simulink model "BugE_v0_40_MAS_loads_reg"  (R2015b)
settings: Solver=FixedStepDiscrete  StartTime=0.0  StopTime=1370  FixedStep=sample_time  RelTol=1e-3
values from neighbouring files (symbols this model uses):
  AB_diode_dV = 0.9    [main_sync.m]
  air_density = 1.225    [main_sync.m]
  bus_ac_Pmax_abs = 240    [main_sync.m]
  bus_charger_Pmax = 1000    [main_sync.m]
  bus_load_Pmax_abs = 260    [main_sync.m]
  capInitVolt = capVmax*sqrt(capInitSoC)    [main_sync.m]
  cyc_kph = [cyc_kph(:,1), cyc_kph(:,2)*speed_max_limit/speed_max]    [main_sync.m]
  cyc_repeat = 0    [main_sync.m]
  ess1_init_soc = 1    [main_sync.m]
  ess1_soh = 1    [main_sync.m]
  ess2_init_soc = 1    [main_sync.m]
  ess2_soh = 1    [main_sync.m]
  ess3_init_soc = 1    [main_sync.m]
  ess3_soh = 1    [main_sync.m]
  ess4_init_soc = 1    [main_sync.m]
  ess4_soh = 1    [main_sync.m]
  ess5_init_soc = 1    [main_sync.m]
  ess5_soh = 1    [main_sync.m]
  gear_ratio = 6    [main_sync.m]
  JADE_on = 0    [main_sync.m]
  loadpower = rawcsv(:,2)    [main_sync.m]
  loadtime = rawcsv(:,1)    [main_sync.m]
  lockSOCs = 0    [main_sync.m]
  max_brk_torque = 300    [main_sync.m]
  no_wheels = 3    [main_sync.m]
  period2 = max(loadtime)    [main_sync.m]
  PV_Pmax = 100    [main_sync.m]
  sample_time = 0.01    [main_sync.m]
  startup_seq_step_delay = 0.2    [main_sync.m]
  stop_option = 0    [main_sync.m]
  use_drive_cycle = 1    [main_sync.m]
  use_real_subs_loads = 1    [main_sync.m]
  vbus_max = 25    [main_sync.m]
  vbus_min = 17    [main_sync.m]
  vbus_safety_threshold = 2    [main_sync.m]
  vbus_threshold = 20    [main_sync.m]
  veh_CD = 0.35    [main_sync.m]
  veh_FA = 1.543    [main_sync.m]
  veh_gravity = 9.81*veh_mass    (= 1863.9)    [main_sync.m]
  veh_mass = 190    [main_sync.m]
  wh_1st_rrc = 0.02    [main_sync.m]
  wh_bearing_frc = 0.0015    [main_sync.m]
  wh_inertia = 0.0556    [main_sync.m]
  wh_radius = 0.508/2    (= 0.254)    [main_sync.m]
undefined symbols (not defined in the file or in its folder): capC, capR, cyc_acc, cyc_avg_time_samples, cyc_brk, cyc_grade, cyc_key, DCM_eff_factor_for_Vin, DCM_eff_for_Iout, DCM_Iout, DCM_Iout_max, DCM_Pin_noload, DCM_Pout_max, DCM_Vin, DCM_Vout, DiscIntNeverNeededParam, ess2_coulombic_eff, ess2_Ineg_max_SOC, ess2_Ineg_max_temp, ess2_Ipos_max_SOC, ess2_Ipos_max_temp, ess2_max_ah_cap, ess2_max_volts, ess2_min_volts, ess2_module_parallel, ess2_module_series, ess2_r_dis, ess2_soc, ess2_SOC_for_Ilimit, ess2_temp_for_Ilimit, ess2_temp_max, ess2_tmp, ess2_voc, ess3_coulombic_eff, ess3_max_ah_cap, ess3_module_parallel, ess3_module_series, ess3_r_dis, ess3_soc, ess3_tmp, ess3_voc, ess_coulombic_eff, ess_Ineg_max_SOC, ess_Ineg_max_temp, ess_Ipos_max_SOC, ess_Ipos_max_temp, ess_max_ah_cap, ess_max_volts, ess_min_volts, ess_module_parallel, ess_module_series, ess_nominal_volts, ess_r_dis, ess_soc, ess_SOC_for_Ilimit, ess_temp_for_Ilimit, ess_temp_max, ess_tmp, ess_voc, MC_eff1 ... (+18)
libraries: simulink x140, commfilt2 x1, simulink_extras x1
(part 2 of 7)

== system BugE_v0_40_MAS_loads_reg/Energy Storage (New Grid)/MB2 DCDC ==
  V batt : Inport
  V bus : Inport  Port=2
  "cmd type 0 P, 1 V " : Inport  Port=3
  cmd value : Inport  Port=4
  I motor : Inport  Port=5
  0 : Constant  Value=eps  SampleTime=sample_time
  Current limiter : Subsystem
  Demux : Demux  Outputs=2
  Demux1 : Demux  Outputs=2
  Demux2 : Demux  Outputs=2
  Energy Quantification : Subsystem
  Imax abs : Constant  Value=MC_Imax  SampleTime=sample_time
  Term : Terminator
  Term1 : Terminator
  V MB nominal : Constant  Value=ess_nominal_volts*ess_module_series  SampleTime=sample_time
  eff_maps : Subsystem
  eff_maps1 : Subsystem
  enabled : Switch  Criteria=u2 > Threshold
  failure mode : Switch  Criteria=u2 > Threshold
  prevent timing errors{,1..3} (4 alike) : UnitDelay  SampleTime=sample_time
  switch2 : Switch  Criteria=u2 > Threshold
  DAB_I_in : Outport
  DAB_I_out : Outport  Port=2
  tag scope: Iin_MB2_DCDC_sensor=global, Iout_MB2_DCDC_sensor=global, Vin_MB2_DCDC=global
  wires:
  Current limiter/2(I bus side lim) -> Energy Quantification/1(In1), DAB_I_out/1, [Iout_MB2_DCDC_sensor]
  Current limiter/1(I batt side lim) -> [Iin_MB2_DCDC_sensor], DAB_I_in/1, Energy Quantification/3(In3)
  V MB nominal/1 -> failure mode/3
  failure mode/1 -> enabled/1
  [RLY_MB] -> prevent timing errors3/1
  [V_MB2_sensor] -> failure mode/1
  Demux/2 -> failure mode/2
  Demux/1 -> Term/1
  Imax abs/1 -> Current limiter/4(I max)
  cmd value/1 -> prevent timing errors2/1
  V batt/1 -> eff_maps/3(Vbatt), Energy Quantification/4(In4)
  V bus/1 -> eff_maps1/3(Vbus), eff_maps/2(Vbus), Energy Quantification/2(In2)
  Demux1/1 -> Current limiter/2(I batt side raw)
  Demux1/2 -> Current limiter/3(I bus side raw)
  "cmd type 0 P, 1 V "/1 -> prevent timing errors1/1
  eff_maps/1(I from batt & into bus) -> switch2/3
  I motor/1 -> eff_maps1/1(I motor)
  switch2/1 -> Demux1/1
  [MB_MOD_PWR] -> prevent timing errors/1
  Demux2/1 -> Term1/1
  enabled/1 -> [Vin_MB2_DCDC]
  0/1 -> enabled/3
  Demux2/2 -> Current limiter/1(enable DCDC), enabled/2
  prevent timing errors/1 -> Demux2/1
  prevent timing errors3/1 -> Demux/1
  prevent timing errors2/1 -> eff_maps1/2(Vbatt cmd), eff_maps/1("P into bus cmd ")
  eff_maps1/1(I from batt & into bus) -> switch2/1
  prevent timing errors1/1 -> switch2/2

== system BugE_v0_40_MAS_loads_reg/Energy Storage (New Grid)/PV_cells Pout ==
  Constant1 : Constant  Value=JADE_on
  Demux : Demux  Outputs=3
  Energy Quantification : Subsystem
  Jade_PW_PV : Constant  Value=[98.16641636677906,1.0,80.83119]  SampleTime=sample_time
  Pmax : Terminator
  Rate Transition24 : RateTransition
  Switch2 : Switch  Criteria=u2 > Threshold
  To Workspace24 : ToWorkspace  VariableName=simout_Level_PV  SampleTime=1
      settings: MaxDataPoints=Inf
  level : Terminator
  power : Outport
  tag scope: PV_Pout_calc=global
  wires:
  [PV_power_lim] -> Switch2/3
  Constant1/1 -> Switch2/2
  Jade_PW_PV/1 -> Demux/1
  Demux/3 -> Switch2/1
  Demux/1 -> Pmax/1
  Demux/2 -> Rate Transition24/1, level/1
  Rate Transition24/1 -> To Workspace24/1
  Switch2/1 -> Energy Quantification/1(Power), [PV_Pout_calc], power/1

== system BugE_v0_40_MAS_loads_reg/Energy Storage (New Grid)/SB1 ==
  Requested power [W] : Inport
  Calculate SOC : Subsystem
  Compute current (nolimit) : Subsystem
  Constant : Constant  Value=0  SampleTime=sample_time
  Demux : Demux  Outputs=2
  Energy Quantification : Subsystem
  "Pack Voc, R" : Subsystem
  Switch : Switch  Criteria=u2 > Threshold
  Terminator : Terminator
  and : Logic  AllPortsSameDT=off  OutDataTypeStr=boolean
  prevent timing errors : UnitDelay  SampleTime=sample_time
  tag scope: SOC_SB1=global, V_SB1_sensor=global
  wires:
  Switch/1 -> Compute current (nolimit)/3(Output power [W]), "Pack Voc, R"/2(Req. power [W])
  Calculate SOC/1(SOC) -> [SOC_SB1]
  "Pack Voc, R"/1(Pack Voc [V]) -> Compute current (nolimit)/1(Voc [V])
  [temp_SB1_sensor] -> "Pack Voc, R"/3(Temp [degC]), Calculate SOC/1(Temp [C])
  [SOC_SB1] -> "Pack Voc, R"/1(SOC_prev)
  "Pack Voc, R"/2(Pack R [Ohm]) -> Energy Quantification/3(In1), Compute current (nolimit)/2(Rint [Ohm])
  Compute current (nolimit)/1(I [A]) -> Energy Quantification/2(In3), Calculate SOC/2(I [A])
  Compute current (nolimit)/2(V [V]) -> Energy Quantification/1(In2), [V_SB1_sensor]
  Constant/1 -> Switch/3
  Requested power [W]/1 -> Switch/1
  Demux/1 -> Switch/2
  Demux/2 -> Terminator/1
  [RLY_SB] -> and/1
  [SB_MOD_PWR] -> and/2
  and/1 -> prevent timing errors/1
  prevent timing errors/1 -> Demux/1

== system BugE_v0_40_MAS_loads_reg/Energy Storage (New Grid)/SB1 DCDC ==
  V batt : Inport
  V bus : Inport  Port=2
  "cmd type 0 P, 1 V " : Inport  Port=3
  cmd value : Inport  Port=4
  Current limiter : Subsystem
  Demux : Demux  Outputs=2
  Demux1 : Demux  Outputs=2
  Energy Quantification : Subsystem
  Imax abs : Constant  Value=MC_Imax  SampleTime=sample_time
  Term : Terminator
  Terminator : Terminator
  eff_maps1 : Subsystem
  enabled : Logic  AllPortsSameDT=off  OutDataTypeStr=boolean
  prevent timing errors : UnitDelay  SampleTime=sample_time
  prevent timing errors1 : UnitDelay  SampleTime=sample_time
  DAB_I_in : Outport
  DAB_I_out : Outport  Port=2
  tag scope: Iin_SB1_DCDC_sensor=global, Iout_SB1_DCDC_sensor=global
  wires:
  Current limiter/2(I bus side lim) -> Energy Quantification/1(In1), DAB_I_out/1, [Iout_SB1_DCDC_sensor]
  Current limiter/1(I batt side lim) -> [Iin_SB1_DCDC_sensor], DAB_I_in/1, Energy Quantification/3(In3)
  Imax abs/1 -> Current limiter/4(I max)
  cmd value/1 -> prevent timing errors1/1
  V batt/1 -> eff_maps1/3(Vbatt), Energy Quantification/4(In4)
  V bus/1 -> eff_maps1/2(Vbus), Energy Quantification/2(In2)
  Demux1/1 -> Current limiter/2(I batt side raw)
  Demux1/2 -> Current limiter/3(I bus side raw)
  eff_maps1/1(I from batt & into bus) -> Demux1/1
  Demux/1 -> prevent timing errors/1
  "cmd type 0 P, 1 V "/1 -> Terminator/1
  enabled/1 -> Demux/1
  Demux/2 -> Term/1
  [SB_MOD_PWR] -> enabled/2
  [RLY_SB] -> enabled/1
  prevent timing errors/1 -> Current limiter/1(enable DCDC)
  prevent timing errors1/1 -> eff_maps1/1("P into bus cmd ")

== system BugE_v0_40_MAS_loads_reg/Energy Storage (New Grid)/SB2 ==
  Requested power [W] : Inport
  Calculate SOC : Subsystem
  Compute current (nolimit) : Subsystem
  Constant : Constant  Value=0  SampleTime=sample_time
  Demux : Demux  Outputs=2
  Energy Quantification : Subsystem
  "Pack Voc, R" : Subsystem
  Switch : Switch  Criteria=u2 > Threshold
  Terminator : Terminator
  and : Logic  AllPortsSameDT=off  OutDataTypeStr=boolean
  prevent timing errors : UnitDelay  SampleTime=sample_time
  tag scope: SOC_SB2=global, V_SB2_sensor=global
  wires:
  Switch/1 -> Compute current (nolimit)/3(Output power [W]), "Pack Voc, R"/2(Req. power [W])
  Calculate SOC/1(SOC) -> [SOC_SB2]
  "Pack Voc, R"/1(Pack Voc [V]) -> Compute current (nolimit)/1(Voc [V])
  [temp_SB2_sensor] -> "Pack Voc, R"/3(Temp [degC]), Calculate SOC/1(Temp [C])
  [SOC_SB2] -> "Pack Voc, R"/1(SOC_prev)
  "Pack Voc, R"/2(Pack R [Ohm]) -> Energy Quantification/3(In1), Compute current (nolimit)/2(Rint [Ohm])
  Compute current (nolimit)/1(I [A]) -> Energy Quantification/2(In3), Calculate SOC/2(I [A])
  Compute current (nolimit)/2(V [V]) -> Energy Quantification/1(In2), [V_SB2_sensor]
  Constant/1 -> Switch/3
  Requested power [W]/1 -> Switch/1
  Demux/2 -> Switch/2
  Demux/1 -> Terminator/1
  [RLY_SB] -> and/1
  [SB_MOD_PWR] -> and/2
  and/1 -> prevent timing errors/1
  prevent timing errors/1 -> Demux/1

== system BugE_v0_40_MAS_loads_reg/Energy Storage (New Grid)/SB2 DCDC ==
  V batt : Inport
  V bus : Inport  Port=2
  "cmd type 0 P, 1 V " : Inport  Port=3
  cmd value : Inport  Port=4
  Current limiter : Subsystem
  Demux : Demux  Outputs=2
  Demux1 : Demux  Outputs=2
  Energy Quantification : Subsystem
  Imax abs : Constant  Value=MC_Imax  SampleTime=sample_time
  Term : Terminator
  Terminator : Terminator
  eff_maps1 : Subsystem
  enabled : Logic  AllPortsSameDT=off  OutDataTypeStr=boolean
  prevent timing errors : UnitDelay  SampleTime=sample_time
  prevent timing errors1 : UnitDelay  SampleTime=sample_time
  DAB_I_in : Outport
  DAB_I_out : Outport  Port=2
  tag scope: Iin_SB2_DCDC_sensor=global, Iout_SB2_DCDC_sensor=global
  wires:
  Current limiter/2(I bus side lim) -> [Iout_SB2_DCDC_sensor], Energy Quantification/1(In1), DAB_I_out/1
  Current limiter/1(I batt side lim) -> [Iin_SB2_DCDC_sensor], DAB_I_in/1, Energy Quantification/3(In3)
  Imax abs/1 -> Current limiter/4(I max)
  cmd value/1 -> prevent timing errors1/1
  V batt/1 -> eff_maps1/3(Vbatt), Energy Quantification/4(In4)
  V bus/1 -> Energy Quantification/2(In2), eff_maps1/2(Vbus)
  Demux1/1 -> Current limiter/2(I batt side raw)
  Demux1/2 -> Current limiter/3(I bus side raw)
  eff_maps1/1(I from batt & into bus) -> Demux1/1
  Demux/2 -> prevent timing errors/1
  "cmd type 0 P, 1 V "/1 -> Terminator/1
  enabled/1 -> Demux/1
  [SB_MOD_PWR] -> enabled/2
  [RLY_SB] -> enabled/1
  Demux/1 -> Term/1
  prevent timing errors/1 -> Current limiter/1(enable DCDC)
  prevent timing errors1/1 -> eff_maps1/1("P into bus cmd ")

== system BugE_v0_40_MAS_loads_reg/Inputs Hardware to Controller/Device detection & identification ==
  note: Modules/Devices detected via CAN communications
  note: Device fault codes from CAN communications
  Constant1 : Constant  SampleTime=sample_time
  Constant2 : Constant  Value=0  SampleTime=sample_time
  Constant3 : Constant  Value=[0,0]  SampleTime=sample_time
  Mux{1..4} (4 alike) : Mux  Inputs=2
  ON_LD : Constant  SampleTime=sample_time
  ON_LDDCDC1 : Constant  SampleTime=sample_time
  ON_MB1 : Constant  SampleTime=sample_time
  ON_MB2 : Constant  SampleTime=sample_time
  ON_SB1 : Constant  SampleTime=sample_time
  ON_SB2 : Constant  SampleTime=sample_time
  tag scope: CHGDCDC_detected=global, CHGDCDC_fcode=global, CHG_detected=global, CHG_fcode=global, LDDCDC_detected=global, LDDCDC_fcode=global, LD_detected=global, LD_fcode=global, MBDCDC_detected=global, MBDCDC_fcode=global, MB_detected=global, MB_fcode=global, PVDCDC_detected=global, PVDCDC_fcode=global, PV_detected=global, PV_fcode=global, SBDCDC_detected=global, SBDCDC_fcode=global, SB_detected=global, SB_fcode=global
  wires:
  Mux1/1 -> [MBDCDC_detected]
  Mux2/1 -> [SBDCDC_detected]
  Mux3/1 -> [SB_detected]
  Mux4/1 -> [MB_detected]
  Constant2/1 -> [PVDCDC_fcode], [CHGDCDC_fcode], [CHG_fcode], [LDDCDC_fcode], [LD_fcode], [PV_fcode]
  Constant3/1 -> [MBDCDC_fcode], [MB_fcode], [SBDCDC_fcode], [SB_fcode]
  Constant1/1 -> [CHG_detected], [CHGDCDC_detected]
  ON_MB1/1 -> Mux1/1, Mux4/1
  ON_SB2/1 -> Mux2/2, Mux3/2
  ON_LDDCDC1/1 -> [PVDCDC_detected], [LDDCDC_detected]
  ON_LD/1 -> [PV_detected], [LD_detected]
  ON_SB1/1 -> Mux2/1, Mux3/1
  ON_MB2/1 -> Mux1/2, Mux4/2

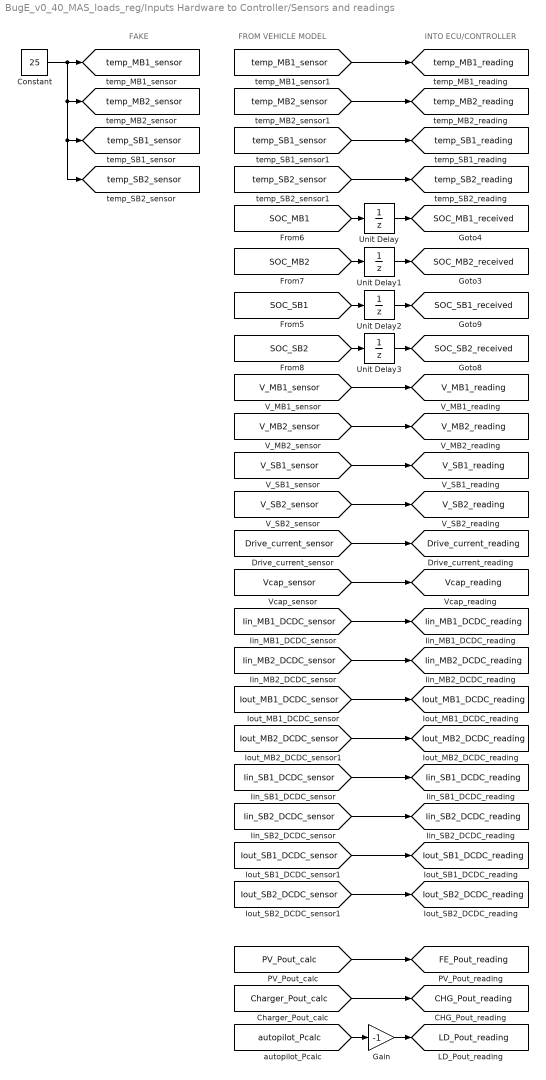
== system BugE_v0_40_MAS_loads_reg/Inputs Hardware to Controller/Sensors and readings ==
  note: FAKE
  note: FROM VEHICLE MODEL
  note: INTO ECU/CONTROLLER
  Constant : Constant  Value=25  SampleTime=sample_time
  Gain : Gain  Gain=-1
  Unit Delay{,1..3} (4 alike) : UnitDelay  InitialCondition=0.9  SampleTime=sample_time
  tag scope: CHG_Pout_reading=global, Drive_current_reading=global, FE_Pout_reading=global, Iin_MB1_DCDC_reading=global, Iin_MB2_DCDC_reading=global, Iin_SB1_DCDC_reading=global, Iin_SB2_DCDC_reading=global, Iout_MB1_DCDC_reading=global, Iout_MB2_DCDC_reading=global, Iout_SB1_DCDC_reading=global, Iout_SB2_DCDC_reading=global, LD_Pout_reading=global, SOC_MB1_received=global, SOC_MB2_received=global, SOC_SB1_received=global, SOC_SB2_received=global, V_MB1_reading=global, V_MB2_reading=global, V_SB1_reading=global, V_SB2_reading=global, Vcap_reading=global, temp_MB1_reading=global, temp_MB1_sensor=global, temp_MB2_reading=global, temp_MB2_sensor=global, temp_SB1_reading=global, temp_SB1_sensor=global, temp_SB2_reading=global, temp_SB2_sensor=global
  wires:
  [Drive_current_sensor] -> [Drive_current_reading]
  [Vcap_sensor] -> [Vcap_reading]
  [V_MB1_sensor] -> [V_MB1_reading]
  [V_MB2_sensor] -> [V_MB2_reading]
  [V_SB1_sensor] -> [V_SB1_reading]
  [V_SB2_sensor] -> [V_SB2_reading]
  [Iout_MB1_DCDC_sensor] -> [Iout_MB1_DCDC_reading]
  [Iout_MB2_DCDC_sensor] -> [Iout_MB2_DCDC_reading]
  [Iin_SB1_DCDC_sensor] -> [Iin_SB1_DCDC_reading]
  [Iout_SB1_DCDC_sensor] -> [Iout_SB1_DCDC_reading]
  [Iin_SB2_DCDC_sensor] -> [Iin_SB2_DCDC_reading]
  [Iout_SB2_DCDC_sensor] -> [Iout_SB2_DCDC_reading]
  Constant/1 -> [temp_MB1_sensor], [temp_SB2_sensor], [temp_SB1_sensor], [temp_MB2_sensor]
  [temp_MB1_sensor] -> [temp_MB1_reading]
  [temp_MB2_sensor] -> [temp_MB2_reading]
  [temp_SB1_sensor] -> [temp_SB1_reading]
  [temp_SB2_sensor] -> [temp_SB2_reading]
  [SOC_MB2] -> Unit Delay1/1
  [SOC_MB1] -> Unit Delay/1
  Unit Delay/1 -> [SOC_MB1_received]
  Unit Delay1/1 -> [SOC_MB2_received]
  [SOC_SB2] -> Unit Delay3/1
  [SOC_SB1] -> Unit Delay2/1
  Unit Delay2/1 -> [SOC_SB1_received]
  Unit Delay3/1 -> [SOC_SB2_received]
  [PV_Pout_calc] -> [FE_Pout_reading]
  [Iin_MB1_DCDC_sensor] -> [Iin_MB1_DCDC_reading]
  [Iin_MB2_DCDC_sensor] -> [Iin_MB2_DCDC_reading]
  [Charger_Pout_calc] -> [CHG_Pout_reading]
  [autopilot_Pcalc] -> Gain/1
  Gain/1 -> [LD_Pout_reading]

== system BugE_v0_40_MAS_loads_reg/Inputs Hardware to Controller/User Inputs ==
  Clock : Clock
  Command Cycles (no regenerative braking assumed) : Subsystem
      mask Display: image('data\images\commands.png')
  Constant : Constant  Value=0  SampleTime=sample_time
  Demux2 : Demux  Outputs=2
  Terminator1 : Terminator
  "key -> ECU bits decode" : Subsystem
  repeat : Constant  Value=cyc_repeat  SampleTime=sample_time
  tag scope: ACC=global, ESTOP=global, IGON=global, throttle=global
  wires:
  Demux2/2 -> Terminator1/1
  Clock/1 -> Command Cycles (no regenerative braking assumed)/2(Time)
  repeat/1 -> Command Cycles (no regenerative braking assumed)/1(repeat)
  "key -> ECU bits decode"/1(ACC) -> [ACC]
  Command Cycles (no regenerative braking assumed)/1(key_out) -> "key -> ECU bits decode"/1(key)
  Demux2/1 -> [throttle]
  "key -> ECU bits decode"/2(IGON) -> [IGON]
  Command Cycles (no regenerative braking assumed)/2(acc_brk_out) -> Demux2/1
  Constant/1 -> [ESTOP]

== system BugE_v0_40_MAS_loads_reg/Inputs Simulation Only/AC load ==
  AC_on : Step  Time=200  Before=1  After=0  SampleTime=sample_time
  AC_power_sine : Gain  Gain=25
  Add : Sum
  Constant : Constant  Value=200  SampleTime=sample_time
  Rate Transition2 : RateTransition
  Saturation : Saturate  UpperLimit=250  LowerLimit=0
  Scope : Scope
  Sine Wave3 : Sin  Frequency=1/2  SampleTime=sample_time
  Switch : Switch  Criteria=u2 > Threshold
  To Workspace3 : ToWorkspace  VariableName=simout_Preq_LD_AC  SampleTime=1
  Zero-Order Hold3 : ZeroOrderHold  SampleTime=sample_time
  off : Constant  Value=0  SampleTime=sample_time
  Out1 : Outport
  wires:
  Zero-Order Hold3/1 -> AC_power_sine/1
  Sine Wave3/1 -> Zero-Order Hold3/1
  AC_power_sine/1 -> Add/1
  Add/1 -> Saturation/1
  Constant/1 -> Add/2
  AC_on/1 -> Switch/2
  Saturation/1 -> Switch/1
  off/1 -> Switch/3
  Switch/1 -> Rate Transition2/1, Scope/1, Out1/1  "A/C"
  Rate Transition2/1 -> To Workspace3/1

== system BugE_v0_40_MAS_loads_reg/Inputs Simulation Only/Autopilot load ==
  Add : Sum
  Constant : Constant  Value=125  SampleTime=sample_time
  Constant2 : Constant  Value=0  SampleTime=sample_time
  Gain : Gain  Gain=0.5
  Look-Up Table3 : Lookup_n-D  NumberOfTableDimensions=1  BreakpointsForDimension1=loadtime(:)  Table=loadpower(:)  ExtrapMethod=Clip  UseLastTableValue=on  InternalRulePriority=Speed  SaturateOnIntegerOverflow=on  InputSameDT=on
  PV_power_sine : Gain  Gain=150
  Rate Transition1 : RateTransition
  Saturation : Saturate  UpperLimit=250  LowerLimit=0
  Saturation1 : Saturate  UpperLimit=245  LowerLimit=0
  Sine Wave3 : Sin  Frequency=1/250  Phase=0.5  SampleTime=sample_time
  Switch : Switch  Criteria=u2 > Threshold
  Switch1 : Switch  Criteria=u2 > Threshold
  To Workspace2 : ToWorkspace  VariableName=simout_Preq_LD_autopilot  SampleTime=1
  Zero-Order Hold3 : ZeroOrderHold  SampleTime=sample_time
  clock w/ pause : Subsystem
  not in standby / startup state : simulink/Logic and Bit Operations/Compare To Constant  relop=>=  const=2  OutDataTypeStr=boolean
  time1 : Fcn  Expr=rem(u,period2)
  use_real_subs_loads : Constant  Value=use_real_subs_loads  SampleTime=sample_time
  Out1 : Outport
  wires:
  Zero-Order Hold3/1 -> PV_power_sine/1
  Sine Wave3/1 -> Zero-Order Hold3/1
  PV_power_sine/1 -> Add/1
  Add/1 -> Saturation/1
  Constant/1 -> Add/2
  Saturation/1 -> Switch/3
  use_real_subs_loads/1 -> Switch/2
  time1/1 -> Look-Up Table3/1
  clock w/ pause/1(Out1) -> time1/1
  Look-Up Table3/1 -> Gain/1
  Switch1/1 -> Switch/1
  [state] -> not in standby / startup state/1
  not in standby / startup state/1 -> clock w/ pause/1(In1), Switch1/2
  Constant2/1 -> Switch1/3
  Gain/1 -> Saturation1/1
  Saturation1/1 -> Switch1/1
  Switch/1 -> Rate Transition1/1, Out1/1  "autopilot"
  Rate Transition1/1 -> To Workspace2/1

== system BugE_v0_40_MAS_loads_reg/Inputs Simulation Only/Auxiliaries power ==
  1: Night 0: Day : Constant  SampleTime=sample_time
  Add : Sum
  Add1 : Sum
  Gain : Gain  Gain=25
  Gain1 : Gain  Gain=35
  Pbus_req : Constant  Value=0  SampleTime=sample_time
  Pbus_req1 : Constant  Value=60  SampleTime=sample_time
  Pulse Generator : DiscretePulseGenerator  PulseType=Time based  Period=10  PulseWidth=30
  Pulse Generator1 : DiscretePulseGenerator  PulseType=Time based  Period=10  PulseWidth=30
  Rate Transition2 : RateTransition
  Scope : Scope
  Switch : Switch  Criteria=u2 > Threshold
  To Workspace3 : ToWorkspace  VariableName=simout_Preq_LD_lights  SampleTime=1
  Out1 : Outport
  wires:
  Add/1 -> Switch/3
  1: Night 0: Day/1 -> Switch/2
  Gain/1 -> Add/1
  Pbus_req/1 -> Add/2
  Add1/1 -> Switch/1
  Pbus_req1/1 -> Add1/2
  Pulse Generator1/1 -> Gain/1
  Pulse Generator/1 -> Gain1/1
  Gain1/1 -> Add1/1
  Switch/1 -> Rate Transition2/1, Scope/1, Out1/1
  Rate Transition2/1 -> To Workspace3/1

== system BugE_v0_40_MAS_loads_reg/Inputs Simulation Only/Charger power ==
  Constant : Constant  Commented=on  Value=100  SampleTime=sample_time
  Constant1 : Constant  Value=300  SampleTime=sample_time
  Discrete-Time Integrator : DiscreteIntegrator  Commented=on  IntegratorMethod=Integration: Trapezoidal  gainval=1  ExternalReset=either  InitialConditionSetting=State (most efficient)  SampleTime=sample_time  LimitOutput=on  UpperSaturationLimit=600  LowerSaturationLimit=0  ICPrevOutput=DiscIntNeverNeededParam  ICPrevScaledInput=DiscIntNeverNeededParam
  Product : Product  Commented=on
  Product1 : Product
  starting time : Step  Commented=on  SampleTime=sample_time
  starting time1 : Step  SampleTime=sample_time
  todouble : DataTypeConversion  Commented=on  OutDataTypeStr=double
  todouble1 : DataTypeConversion  OutDataTypeStr=double
  Out1 : Outport
  wires:
  todouble/1 -> Product/2
  Constant/1 -> Discrete-Time Integrator/1
  Discrete-Time Integrator/1 -> Product/1
  starting time/1 -> Discrete-Time Integrator/2, todouble/1
  todouble1/1 -> Product1/2
  starting time1/1 -> todouble1/1
  Product1/1 -> Out1/1
  Constant1/1 -> Product1/1

== system BugE_v0_40_MAS_loads_reg/Inputs Simulation Only/Command Cycles ==
  repeat : Inport
  Time : Inport  Port=2
  Constant : Constant  Value=max(cyc_key(:,1))  SampleTime=sample_time
  Demux2 : Demux  Outputs=2
  From Workspace1 : FromWorkspace  VariableName=cyc_grade_ts  SampleTime=sample_time
  Look-Up Table1 : Lookup_n-D  NumberOfTableDimensions=1  BreakpointsForDimension1=cyc_grade(:,1)  Table=cyc_grade(:,2)  InternalRulePriority=Speed  SaturateOnIntegerOverflow=on  InputSameDT=on
  Rate Limiter 0-full in 1s : RateLimiter  SampleTimeMode=inherited
  Relational Operator : RelationalOperator  OutDataTypeStr=boolean
  Scope : Scope
  Switch1 : Switch  Criteria=u2 > Threshold
  Switch2 : Switch  Criteria=u2 > Threshold
  Terminator1 : Terminator
  Terminator2 : Terminator
  drive_cycle : Subsystem
  key : Subsystem
  pedal cycle : Subsystem
  source : Switch  Criteria=u2 > Threshold
  time : Fcn  Expr=rem(u,period)
  use_drive_cycle : Constant  Value=use_drive_cycle  SampleTime=sample_time
  zero : Constant  Value=0  SampleTime=sample_time
  acc_brk_out : Outport
  endcycle_stopsim : Outport  Port=2
  grade : Outport  Port=3
  wires:
  time/1 -> Look-Up Table1/1, drive_cycle/1(time), pedal cycle/2(time), key/1(time)
  Look-Up Table1/1 -> Switch1/1
  From Workspace1/1 -> Switch1/3
  Switch1/1 -> grade/1  "grade"
  zero/1 -> Switch2/1
  Relational Operator/1 -> Switch2/3
  Time/1 -> Relational Operator/1, time/1
  Constant/1 -> Relational Operator/2
  repeat/1 -> key/2(repeat), Switch2/2, Switch1/2, drive_cycle/2(repeat), pedal cycle/3(repeat)
  source/1 -> Rate Limiter 0-full in 1s/1
  key/2(motor_on) -> pedal cycle/1(motor_on)
  use_drive_cycle/1 -> source/2
  pedal cycle/1(acc/brk) -> source/3
  drive_cycle/1(acc/brk) -> source/1
  [velocity_kph] -> drive_cycle/3(velocity kph)
  Switch2/1 -> endcycle_stopsim/1
  key/1(key) -> Terminator2/1  "key position"
  Rate Limiter 0-full in 1s/1 -> Demux2/1  "acc, brk"
  Demux2/1 -> Terminator1/1
  Demux2/2 -> Scope/1, acc_brk_out/1

== system BugE_v0_40_MAS_loads_reg/Inputs Simulation Only/PV power ==
  Band-Limited White Noise2 : simulink/Sources/Band-Limited White Noise  Cov=[0.025]  Ts=sample_time  seed=[23341]
  PV_power : Sum  Inputs=+++
  PV_power_base : Constant  Value=85  SampleTime=sample_time
  PV_power_sine : Gain  Gain=5
  Product : Product
  Sine Wave3 : Sin  Frequency=1/5  SampleTime=sample_time
  Zero-Order Hold3 : ZeroOrderHold  SampleTime=sample_time
  Zero-Order Hold4 : ZeroOrderHold  SampleTime=sample_time
  step: starting time : Step  Time=175  SampleTime=sample_time
  Out1 : Outport
  wires:
  Product/1 -> Out1/1
  PV_power_sine/1 -> PV_power/2
  Zero-Order Hold3/1 -> PV_power_sine/1
  PV_power/1 -> Product/2
  Band-Limited White Noise2/1 -> PV_power/3
  step: starting time/1 -> Zero-Order Hold4/1
  Sine Wave3/1 -> Zero-Order Hold3/1
  Zero-Order Hold4/1 -> Product/1
  PV_power_base/1 -> PV_power/1

== system BugE_v0_40_MAS_loads_reg/Inputs Simulation Only/Standby load ==
  Add : Sum  Inputs=++++
  Band-Limited White Noise : simulink/Sources/Band-Limited White Noise  Cov=[0.0025]  Ts=sample_time  seed=[23341]
  Gain1 : Gain  Gain=2
  Gain2 : Gain  Gain=4
  Pbus_req1 : Constant  Value=8.2  SampleTime=sample_time
  Sine Wave1 : Sin  SampleTime=sample_time
  Sine Wave2 : Sin  Frequency=1/50  SampleTime=sample_time
  Switch : Switch  Criteria=u2 > Threshold
  Zero-Order Hold : ZeroOrderHold  SampleTime=sample_time
  Zero-Order Hold1 : ZeroOrderHold  SampleTime=sample_time
  use_real_subs_loads : Constant  Value=use_real_subs_loads  SampleTime=sample_time
  Out1 : Outport
  wires:
  Sine Wave1/1 -> Zero-Order Hold1/1
  Zero-Order Hold/1 -> Gain2/1
  Sine Wave2/1 -> Zero-Order Hold/1
  Zero-Order Hold1/1 -> Gain1/1
  Gain2/1 -> Add/2
  Gain1/1 -> Add/3
  Band-Limited White Noise/1 -> Add/4
  Add/1 -> Switch/3
  use_real_subs_loads/1 -> Switch/2
  Switch/1 -> Out1/1
  Pbus_req1/1 -> Add/1, Switch/1

== system BugE_v0_40_MAS_loads_reg/Inputs Simulation Only/USB power ==
  Gain : Gain  Gain=12
  Rate Transition2 : RateTransition
  Switch : Switch  Criteria=u2 > Threshold
  To Workspace3 : ToWorkspace  VariableName=simout_Preq_LD_USB  SampleTime=1
  USB ports on : Step  Time=10000  SampleTime=sample_time
  USB1 : Constant  Value=2
  off : Constant  Value=0
  Out1 : Outport
  wires:
  USB1/1 -> Gain/1
  Switch/1 -> Rate Transition2/1, Out1/1
  Gain/1 -> Switch/1
  off/1 -> Switch/3
  USB ports on/1 -> Switch/2
  Rate Transition2/1 -> To Workspace3/1

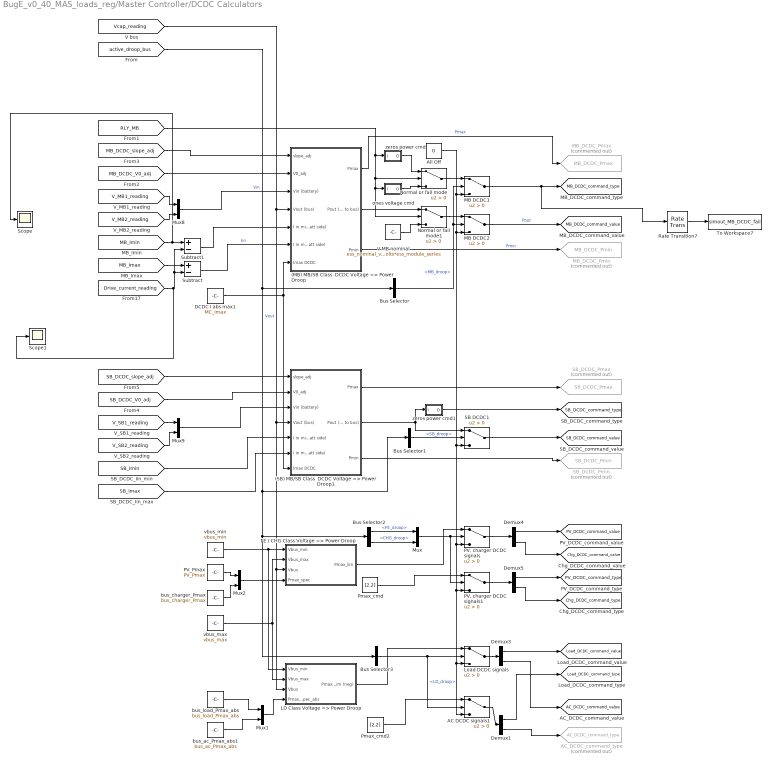
== system BugE_v0_40_MAS_loads_reg/Master Controller/DCDC Calculators ==
  (MB) MB/SB Class  DCDC Voltage => Power Droop : Subsystem
  (SB) MB/SB Class  DCDC Voltage => Power Droop1 : Subsystem
  AC DCDC signals1 : Switch  Criteria=u2 > Threshold
  AC_DCDC_command_type : Goto  Commented=on  GotoTag=AC_DCDC_command_type  TagVisibility=global
  All Off : Constant  Value=0  SampleTime=sample_time
  Bus Selector : BusSelector  OutputSignals=MB_droop
  Bus Selector1 : BusSelector  OutputSignals=SB_droop
  Bus Selector2 : BusSelector  OutputSignals=FE_droop,CHG_droop
  Bus Selector3 : BusSelector  OutputSignals=LD_droop
  DCDC I abs max1 : Constant  Value=MC_Imax  SampleTime=sample_time
  Demux{1,3..5} (4 alike) : Demux  Outputs=2
  FE / CHG Class Voltage => Power Droop : Subsystem
  LD Class Voltage => Power Droop : Subsystem
  Load DCDC signals : Switch  Criteria=u2 > Threshold
  MB DCDC1 : Switch  Criteria=u2 > Threshold
  MB DCDC2 : Switch  Criteria=u2 > Threshold
  MB_DCDC_Pmax : Goto  Commented=on  GotoTag=MB_DCDC_Pmax  TagVisibility=global
  MB_DCDC_Pmin : Goto  Commented=on  GotoTag=MB_DCDC_Pmin  TagVisibility=global
  Mux{,1..2,8..9} (5 alike) : Mux  Inputs=2
  Normal or fail mode : Switch  Criteria=u2 > Threshold
  Normal or fail mode1 : Switch  Criteria=u2 > Threshold
  "PV, charger DCDC signals" : Switch  Criteria=u2 > Threshold
  "PV, charger DCDC signals1" : Switch  Criteria=u2 > Threshold
  PV_Pmax : Constant  Value=PV_Pmax  SampleTime=sample_time
  Pmax_cmd : Constant  Value=[2,2]  SampleTime=sample_time
  Pmax_cmd2 : Constant  Value=[2,2]  SampleTime=sample_time
  Rate Transition7 : RateTransition
  SB DCDC1 : Switch  Criteria=u2 > Threshold
  SB_DCDC_Pmax : Goto  Commented=on  GotoTag=SB_DCDC_Pmax  TagVisibility=global
  SB_DCDC_Pmin : Goto  Commented=on  GotoTag=SB_DCDC_Pmin  TagVisibility=global
  Scope : Scope
  Scope1 : Scope
  Subtract : Sum  Inputs=+-
  Subtract1 : Sum  Inputs=+-
  To Workspace7 : ToWorkspace  VariableName=simout_MB_DCDC_fail  SampleTime=1
  V MB nominal : Constant  Value=ess_nominal_volts*ess_module_series  SampleTime=sample_time
  bus_ac_Pmax_abs1 : Constant  Value=bus_ac_Pmax_abs  SampleTime=sample_time
  bus_charger_Pmax : Constant  Value=bus_charger_Pmax  SampleTime=sample_time
  bus_load_Pmax_abs : Constant  Value=bus_load_Pmax_abs  SampleTime=sample_time
  ones voltage cmd : Subsystem
  vbus_max : Constant  Value=vbus_max  SampleTime=sample_time
  vbus_min : Constant  Value=vbus_min  SampleTime=sample_time
  zeros power cmd : Subsystem
  zeros power cmd1 : Subsystem
  tag scope: AC_DCDC_command_value=global, Chg_DCDC_command_type=global, Chg_DCDC_command_value=global, Load_DCDC_command_type=global, Load_DCDC_command_value=global, MB_DCDC_command_type=global, MB_DCDC_command_value=global, PV_DCDC_command_type=global, PV_DCDC_command_value=global, SB_DCDC_command_type=global, SB_DCDC_command_value=global
  wires:
  vbus_min/1 -> LD Class Voltage => Power Droop/1(Vbus_min), FE / CHG Class Voltage => Power Droop/1(Vbus_min)
  vbus_max/1 -> LD Class Voltage => Power Droop/2(Vbus_max), FE / CHG Class Voltage => Power Droop/2(Vbus_max)
  Mux8/1 -> (MB) MB/SB Class  DCDC Voltage => Power Droop/3(Vin (battery))  "Vin"
  Mux9/1 -> (SB) MB/SB Class  DCDC Voltage => Power Droop1/3(Vin (battery))
  [RLY_MB] -> Normal or fail mode1/2, ones voltage cmd/1(I), Normal or fail mode/2, zeros power cmd/1(I)
  ones voltage cmd/1(O) -> Normal or fail mode/3
  zeros power cmd/1(O) -> Normal or fail mode/1
  (MB) MB/SB Class  DCDC Voltage => Power Droop/2(Pout (MC to bus)) -> Normal or fail mode1/1
  All Off/1 -> "PV, charger DCDC signals1"/3, AC DCDC signals1/3, Load DCDC signals/3, "PV, charger DCDC signals"/3, SB DCDC1/3, MB DCDC2/3, MB DCDC1/3
  Normal or fail mode/1 -> MB DCDC1/1
  V MB nominal/1 -> Normal or fail mode1/3
  PV_Pmax/1 -> Mux2/1
  bus_charger_Pmax/1 -> Mux2/2
  Mux2/1 -> FE / CHG Class Voltage => Power Droop/4(Pmax_spec)
  Mux/1 -> "PV, charger DCDC signals"/2, "PV, charger DCDC signals1"/2
  FE / CHG Class Voltage => Power Droop/1(Pmax_lim) -> "PV, charger DCDC signals"/1
  Load DCDC signals/1 -> Demux3/1
  "PV, charger DCDC signals"/1 -> Demux4/1
  Demux4/1 -> [PV_DCDC_command_value]
  Demux4/2 -> [Chg_DCDC_command_value]
  Demux5/1 -> [PV_DCDC_command_type]
  Demux5/2 -> [Chg_DCDC_command_type]
  Demux3/1 -> [Load_DCDC_command_value]
  [active_droop_bus] -> Bus Selector2/1, Bus Selector3/1, Bus Selector1/1, Bus Selector/1
  [SB_Imin] -> (SB) MB/SB Class  DCDC Voltage => Power Droop1/5(I in min (batt side))
  [SB_Imax] -> (SB) MB/SB Class  DCDC Voltage => Power Droop1/6(I in max (batt side))
  DCDC I abs max1/1 -> (SB) MB/SB Class  DCDC Voltage => Power Droop1/7(Imax DCDC), (MB) MB/SB Class  DCDC Voltage => Power Droop/7(Imax DCDC)
  (SB) MB/SB Class  DCDC Voltage => Power Droop1/2(Pout (MC to bus)) -> zeros power cmd1/1(I), SB DCDC1/1
  Bus Selector1/1 -> SB DCDC1/2  "<SB_droop>"
  zeros power cmd1/1(O) -> [SB_DCDC_command_type]
  Normal or fail mode1/1 -> MB DCDC2/1
  "PV, charger DCDC signals1"/1 -> Demux5/1
  Pmax_cmd/1 -> "PV, charger DCDC signals1"/1
  Bus Selector/1 -> MB DCDC1/2, MB DCDC2/2  "<MB_droop>"
  [V_MB1_reading] -> Mux8/1
  [V_MB2_reading] -> Mux8/2
  [V_SB1_reading] -> Mux9/1
  [V_SB2_reading] -> Mux9/2
  Bus Selector2/2 -> Mux/2  "<CHG_droop>"
  Bus Selector2/1 -> Mux/1  "<FE_droop>"
  Bus Selector3/1 -> AC DCDC signals1/2, Load DCDC signals/2  "<LD_droop>"
  Subtract/1 -> (MB) MB/SB Class  DCDC Voltage => Power Droop/6(I in max (batt side))  "Iin"
  [MB_Imin] -> Scope/1, Subtract1/1
  [MB_Imax] -> Subtract/1
  [MB_DCDC_V0_adj] -> (MB) MB/SB Class  DCDC Voltage => Power Droop/2(V0_adj)
  [MB_DCDC_slope_adj] -> (MB) MB/SB Class  DCDC Voltage => Power Droop/1(slope_adj)
  [SB_DCDC_V0_adj] -> (SB) MB/SB Class  DCDC Voltage => Power Droop1/2(V0_adj)
  [SB_DCDC_slope_adj] -> (SB) MB/SB Class  DCDC Voltage => Power Droop1/1(slope_adj)
  MB DCDC1/1 -> Rate Transition7/1, [MB_DCDC_command_type]
  SB DCDC1/1 -> [SB_DCDC_command_value]
  (MB) MB/SB Class  DCDC Voltage => Power Droop/1(" Pmax ") -> MB_DCDC_Pmax/1  "Pmax"
  (MB) MB/SB Class  DCDC Voltage => Power Droop/3(" Pmin ") -> MB_DCDC_Pmin/1  "Pmin"
  [Vcap_reading] -> (SB) MB/SB Class  DCDC Voltage => Power Droop1/4(Vout (bus)), FE / CHG Class Voltage => Power Droop/3(Vbus), LD Class Voltage => Power Droop/3(Vbus), (MB) MB/SB Class  DCDC Voltage => Power Droop/4(Vout (bus))  "Vout"
  MB DCDC2/1 -> [MB_DCDC_command_value]  "Pout"
  (SB) MB/SB Class  DCDC Voltage => Power Droop1/1(" Pmax ") -> SB_DCDC_Pmax/1
  (SB) MB/SB Class  DCDC Voltage => Power Droop1/3(" Pmin") -> SB_DCDC_Pmin/1
  Rate Transition7/1 -> To Workspace7/1
  Mux1/1 -> LD Class Voltage => Power Droop/4(Pmax_spec_abs)
  bus_load_Pmax_abs/1 -> Mux1/1
  bus_ac_Pmax_abs1/1 -> Mux1/2
  Demux3/2 -> [AC_DCDC_command_value]
  LD Class Voltage => Power Droop/1(Pmax_lim (neg)) -> Load DCDC signals/1
  Pmax_cmd2/1 -> AC DCDC signals1/1
  AC DCDC signals1/1 -> Demux1/1
  Demux1/2 -> AC_DCDC_command_type/1
  Demux1/1 -> [Load_DCDC_command_type]
  Subtract1/1 -> (MB) MB/SB Class  DCDC Voltage => Power Droop/5(I in min (batt side))
  [Drive_current_reading] -> Scope1/1, Subtract1/2, Subtract/2

== system BugE_v0_40_MAS_loads_reg/Master Controller/Detection ==
  Bus Creator : BusCreator  Inputs=10
  Bus Selector1 : BusSelector  OutputSignals=MB MOD PWR,SB_MOD_PWR,FE_MOD_PWR,CHG_MOD_PWR,LD_MOD_PWR
  Unit Delay1 : UnitDelay  SampleTime=sample_time
  and{,1..9} (10 alike) : Logic  AllPortsSameDT=off  OutDataTypeStr=boolean
  tag scope: devices_ON_bus=global
  wires:
  and5/1 -> Bus Creator/6  "MB_on"
  and7/1 -> Bus Creator/8  "FE_on"
  and6/1 -> Bus Creator/7  "SB_on"
  and3/1 -> Bus Creator/4  "CHGDCDC_on"
  and2/1 -> Bus Creator/3  "FEDCDC_on"
  and8/1 -> Bus Creator/9  "CHG_on"
  and9/1 -> Bus Creator/10  "LD_on"
  and4/1 -> Bus Creator/5  "LDDCDC_on"
  and1/1 -> Bus Creator/2  "SBDCDC_on"
  and/1 -> Bus Creator/1  "MBDCDC_on"
  Bus Creator/1 -> [devices_ON_bus]
  [MBDCDC_detected] -> and/1
  [PVDCDC_detected] -> and2/1
  [CHGDCDC_detected] -> and3/1
  [LDDCDC_detected] -> and4/1
  [MB_detected] -> and5/1
  [SB_detected] -> and6/1
  [PV_detected] -> and7/1
  [CHG_detected] -> and8/1
  [LD_detected] -> and9/1
  [SBDCDC_detected] -> and1/1
  [device_power_on_bus] -> Unit Delay1/1
  Unit Delay1/1 -> Bus Selector1/1
  Bus Selector1/1 -> and/2, and5/2  "<MB MOD PWR>"
  Bus Selector1/2 -> and6/2, and1/2  "<SB_MOD_PWR>"
  Bus Selector1/3 -> and7/2, and2/2  "<FE_MOD_PWR>"
  Bus Selector1/4 -> and3/2, and8/2  "<CHG_MOD_PWR>"
  Bus Selector1/5 -> and4/2, and9/2  "<LD_MOD_PWR>"

== system BugE_v0_40_MAS_loads_reg/Master Controller/Motor Controller ==
  "1 if relay closed, 0 if relay open" : DataTypeConversion  OutDataTypeStr=double
  Constant1 : Constant  Value=0  SampleTime=sample_time
  Iout_MB1 : Sum
  Iout_MB2 : Sum
  MB Class Current => Throttle Droop : Subsystem
  MB DCDC Imax : Constant  Value=MC_Imax  SampleTime=sample_time
  Motor Imax : Constant  Value=mc_max_crrnt  SampleTime=sample_time
  Saturation Dynamic : simulink/Discontinuities/Saturation Dynamic  OutMin=[]  OutMax=[]  OutDataTypeStr=Inherit: Same as second input  OutDataType=fixdt(1, 16)  OutScaling=2^-10  DoSatur=off
  Switch : Switch  Criteria=u2 > Threshold
  largest current read : MinMax  Function=max  Inputs=2
  min : MinMax  Inputs=2
  min1 : MinMax
  smallest maximum current : MinMax  Inputs=2
  tag scope: throttle_adjusted=global
  wires:
  [Drive_current_reading] -> Iout_MB2/1, Iout_MB1/1
  [Iin_MB1_DCDC_reading] -> Iout_MB1/2
  [Iin_MB2_DCDC_reading] -> Iout_MB2/2
  Iout_MB1/1 -> largest current read/1
  Iout_MB2/1 -> largest current read/2
  [RLY_MB] -> Switch/2
  MB DCDC Imax/1 -> Switch/3
  smallest maximum current/1 -> MB Class Current => Throttle Droop/2(Imax)
  largest current read/1 -> MB Class Current => Throttle Droop/1(I)
  Constant1/1 -> Saturation Dynamic/3
  min/1 -> Saturation Dynamic/1
  [RLY_DRV] -> "1 if relay closed, 0 if relay open"/1
  "1 if relay closed, 0 if relay open"/1 -> min/1
  MB Class Current => Throttle Droop/1(thr_max_lim) -> min/2  "ems_MC_thr_droop"
  min1/1 -> smallest maximum current/2
  Motor Imax/1 -> smallest maximum current/1
  Saturation Dynamic/1 -> [throttle_adjusted]
  [throttle] -> Saturation Dynamic/2
  [MB_Imax] -> Switch/1
  Switch/1 -> min1/1

== system BugE_v0_40_MAS_loads_reg/Master Controller/Operating Mode Controller ==
  Accessories (State 2) : Subsystem  TreatAsAtomicUnit=on
  Driving (State 3) : Subsystem  TreatAsAtomicUnit=on
  SM flags : Scope  NumInputPorts=4
  Scope : Scope
  Standby (State 0) : Subsystem  TreatAsAtomicUnit=on
  Startup sequence (State 1) : Subsystem  TreatAsAtomicUnit=on
  "State machine 0 std, 1 startup, 2 acc, 3 drv, 4 fault" : Subsystem
  bus charged & within limits : Subsystem
  ready for driving : Subsystem
  start-up ready : Subsystem
  tag scope: RLYs_and_12V_bus2=global, RLYs_and_12V_bus3=global, RLYs_and_12V_bus4=global, RLYs_and_12V_bus=global, SM_SUR_flag=global, droop_bus2=global, droop_bus3=global, droop_bus4=global, droop_bus=global, module_PWR_bus2=global, module_PWR_bus=global, state=global
  wires:
  "State machine 0 std, 1 startup, 2 acc, 3 drv, 4 fault"/3(enable_startup) -> Startup sequence (State 1)/Enable
  "State machine 0 std, 1 startup, 2 acc, 3 drv, 4 fault"/5(enable_driving) -> Driving (State 3)/Enable
  "State machine 0 std, 1 startup, 2 acc, 3 drv, 4 fault"/2(enable_standby) -> Standby (State 0)/Enable
  Standby (State 0)/1(RLYs_and_12V bus) -> [RLYs_and_12V_bus]
  Standby (State 0)/2(module_PWR bus) -> [module_PWR_bus]
  Standby (State 0)/3(droop_bus) -> [droop_bus]
  bus charged & within limits/1(bus_ready) -> Startup sequence (State 1)/2(bus ready)
  Accessories (State 2)/2(droop_bus) -> [droop_bus3]
  "State machine 0 std, 1 startup, 2 acc, 3 drv, 4 fault"/4(enable_accessories) -> Accessories (State 2)/Enable
  [devices_ON_bus] -> Standby (State 0)/1(devices_ON bus), Startup sequence (State 1)/1(devices_ON bus), Driving (State 3)/1(devices_ON bus), Accessories (State 2)/1(devices_ON bus)
  Startup sequence (State 1)/2(droop_bus) -> [droop_bus2]
  Startup sequence (State 1)/3(SUR) -> [SM_SUR_flag]
  Driving (State 3)/2(droop_bus) -> [droop_bus4]
  Startup sequence (State 1)/1(RLYs_and_12V bus) -> [RLYs_and_12V_bus2]
  Startup sequence (State 1)/4(module_PWR bus) -> [module_PWR_bus2]
  Accessories (State 2)/1(RLYs_and_12V bus) -> [RLYs_and_12V_bus3]
  Driving (State 3)/1(RLYs_and_12V bus) -> [RLYs_and_12V_bus4]
  [ESTOP] -> "State machine 0 std, 1 startup, 2 acc, 3 drv, 4 fault"/5(ESTOP (user triggered e-stop))
  "State machine 0 std, 1 startup, 2 acc, 3 drv, 4 fault"/1(state) -> [state], Scope/1  "ems_SM_state"
  [ACC] -> SM flags/3, "State machine 0 std, 1 startup, 2 acc, 3 drv, 4 fault"/1(ACC)
  ready for driving/1(RFD) -> SM flags/1, "State machine 0 std, 1 startup, 2 acc, 3 drv, 4 fault"/3(RFD (ready for driving))  "RFD"
  start-up ready/1(SUR) -> SM flags/2, "State machine 0 std, 1 startup, 2 acc, 3 drv, 4 fault"/4(SUR (startup ready))  "SUR"
  [IGON] -> SM flags/4, "State machine 0 std, 1 startup, 2 acc, 3 drv, 4 fault"/2(IGON)

== system BugE_v0_40_MAS_loads_reg/Master Controller/Secondary Objectives ==
  MB SOC balancing : Subsystem
  Motor MBDCDC boost : Subsystem
  Scope : Scope  NumInputPorts=4
  Source prioritization : Subsystem
  Switch : Switch  Criteria=u2 > Threshold
  boosting : simulink/Logic and Bit Operations/Compare To Zero  relop=~=  OutDataTypeStr=boolean
  enable_balancing : Constant  SampleTime=sample_time
  enable_boost : Constant  Value=0  SampleTime=sample_time
  enable_prioritization : Constant  SampleTime=sample_time
  tag scope: MB_DCDC_V0_adj=global, MB_DCDC_slope_adj=global, SB_DCDC_V0_adj=global, SB_DCDC_slope_adj=global
  wires:
  enable_boost/1 -> Motor MBDCDC boost/1(enable)
  enable_prioritization/1 -> Source prioritization/1(enable)
  enable_balancing/1 -> MB SOC balancing/1(enable)
  MB SOC balancing/1(MB slope adj) -> [MB_DCDC_slope_adj], Scope/1  "MB_DCDC_slope_adj"
  Switch/1 -> [MB_DCDC_V0_adj], Scope/3  "MB_DCDC_V0_adj"
  Source prioritization/3(SB V0 adj) -> [SB_DCDC_V0_adj], Scope/4  "SB_DCDC_V0_adj"
  Source prioritization/1(SB slope adj) -> [SB_DCDC_slope_adj], Scope/2  "SB_DCDC_slope_adj"
  boosting/1 -> Switch/2
  Motor MBDCDC boost/1(MB V0 adj) -> Switch/1, boosting/1
  Source prioritization/2(MB V0 adj) -> Switch/3

== system BugE_v0_40_MAS_loads_reg/Master Controller/Signal Buffer ==
  (0 device OFF / 1 ON)1 : Subsystem
  (0 device OFF / 1 ON)10 : Subsystem
  (0 device OFF / 1 ON)11 : Subsystem
  (0 device OFF / 1 ON)12 : Subsystem
  (0 device OFF / 1 ON)13 : Subsystem
  (0 device OFF / 1 ON)14 : Subsystem
  (0 device OFF / 1 ON)15 : Subsystem
  (0 device OFF / 1 ON)16 : Subsystem
  (0 device OFF / 1 ON)2 : Subsystem
  (0 device OFF / 1 ON)3 : Subsystem
  (0 device OFF / 1 ON)4 : Subsystem
  (0 device OFF / 1 ON)5 : Subsystem
  (0 device OFF / 1 ON)6 : Subsystem
  (0 device OFF / 1 ON)7 : Subsystem
  (0 device OFF / 1 ON)8 : Subsystem
  (0 device OFF / 1 ON)9 : Subsystem
  Bus Creator : BusCreator  Inputs=5
  Bus Creator1 : BusCreator  Inputs=5
  Bus Selector1 : BusSelector  OutputSignals=MB_MOD_PWR_EN,MB_MOD_PWR_DSBL,SB_MOD_PWR_EN,SB_MOD_PWR_DSBL,FE_PWR_EN,FE_PWR_DSBL,CHG_PWR_EN,CHG_PWR_DSBL,LD_PWR_EN,LD_PWR_DSBL
  Bus Selector2 : BusSelector  OutputSignals=MB_droop_EN,MB_droop_DSBL,SB_droop_EN,SB_droop_DSBL,FE_droop_EN,FE_droop_DSBL,CHG_droop_EN,CHG_droop_DSBL,LD_droop_EN,LD_droop_DSBL
  Bus Selector5 : BusSelector  OutputSignals=RLY_MB_EN,RLY_MB_DSBL,RLY_SB_EN,RLY_SB_DSBL,RLY_AUX_EN,RLY_AUX_DSBL,RLY_DRV_EN,RLY_DRV_DSBL,RLY_EDLC_EN,RLY_EDLC_DSBL,DDC_EN,DDC_DSBL
  Goto11 : Goto  Commented=on  GotoTag=LD_MOD_PWR  TagVisibility=global
  Goto3 : Goto  Commented=on  GotoTag=FE_MOD_PWR  TagVisibility=global
  Goto6 : Goto  Commented=on  GotoTag=CHG_MOD_PWR  TagVisibility=global
  RLYs_and_12V_bus : Subsystem
  droop_bus : Subsystem
  module_PWR_bus : Subsystem
  tag scope: DDC=global, MB_MOD_PWR=global, RLY_AUX=global, RLY_DRV=global, RLY_EDLC=global, RLY_MB=global, RLY_SB=global, SB_MOD_PWR=global, active_droop_bus=global, device_power_on_bus=global
  wires:
  (0 device OFF / 1 ON)7/1(state) -> Bus Creator1/1, [MB_MOD_PWR]  "MB MOD PWR"
  RLYs_and_12V_bus/1(Out1) -> Bus Selector5/1
  module_PWR_bus/1(Out1) -> Bus Selector1/1
  droop_bus/1(Out1) -> Bus Selector2/1
  Bus Selector5/1 -> (0 device OFF / 1 ON)10/1(EN)  "<RLY_MB_EN>"
  Bus Selector5/2 -> (0 device OFF / 1 ON)10/2(DSBL)  "<RLY_MB_DSBL>"
  Bus Selector5/3 -> (0 device OFF / 1 ON)1/1(EN)  "<RLY_SB_EN>"
  Bus Selector5/4 -> (0 device OFF / 1 ON)1/2(DSBL)  "<RLY_SB_DSBL>"
  Bus Selector5/5 -> (0 device OFF / 1 ON)3/1(EN)  "<RLY_AUX_EN>"
  Bus Selector5/6 -> (0 device OFF / 1 ON)3/2(DSBL)  "<RLY_AUX_DSBL>"
  Bus Selector5/7 -> (0 device OFF / 1 ON)2/1(EN)  "<RLY_DRV_EN>"
  Bus Selector5/8 -> (0 device OFF / 1 ON)2/2(DSBL)  "<RLY_DRV_DSBL>"
  Bus Selector5/9 -> (0 device OFF / 1 ON)5/1(EN)  "<RLY_EDLC_EN>"
  Bus Selector5/10 -> (0 device OFF / 1 ON)5/2(DSBL)  "<RLY_EDLC_DSBL>"
  Bus Selector5/11 -> (0 device OFF / 1 ON)4/1(EN)  "<DDC_EN>"
  Bus Selector5/12 -> (0 device OFF / 1 ON)4/2(DSBL)  "<DDC_DSBL>"
  (0 device OFF / 1 ON)10/1(state) -> [RLY_MB]
  (0 device OFF / 1 ON)1/1(state) -> [RLY_SB]
  (0 device OFF / 1 ON)3/1(state) -> [RLY_AUX]
  (0 device OFF / 1 ON)2/1(state) -> [RLY_DRV]
  (0 device OFF / 1 ON)5/1(state) -> [RLY_EDLC]
  (0 device OFF / 1 ON)4/1(state) -> [DDC]
  Bus Selector1/2 -> (0 device OFF / 1 ON)7/2(DSBL)  "<MB_MOD_PWR_DSBL>"
  Bus Selector1/1 -> (0 device OFF / 1 ON)7/1(EN)  "<MB_MOD_PWR_EN>"
  Bus Selector1/4 -> (0 device OFF / 1 ON)6/2(DSBL)  "<SB_MOD_PWR_DSBL>"
  Bus Selector1/3 -> (0 device OFF / 1 ON)6/1(EN)  "<SB_MOD_PWR_EN>"
  Bus Selector1/6 -> (0 device OFF / 1 ON)9/2(DSBL)  "<FE_PWR_DSBL>"
  Bus Selector1/5 -> (0 device OFF / 1 ON)9/1(EN)  "<FE_PWR_EN>"
  Bus Selector1/8 -> (0 device OFF / 1 ON)8/2(DSBL)  "<CHG_PWR_DSBL>"
  Bus Selector1/7 -> (0 device OFF / 1 ON)8/1(EN)  "<CHG_PWR_EN>"
  Bus Selector1/10 -> (0 device OFF / 1 ON)11/2(DSBL)  "<LD_PWR_DSBL>"
  Bus Selector1/9 -> (0 device OFF / 1 ON)11/1(EN)  "<LD_PWR_EN>"
  (0 device OFF / 1 ON)6/1(state) -> Bus Creator1/2, [SB_MOD_PWR]  "SB_MOD_PWR"
  (0 device OFF / 1 ON)9/1(state) -> Bus Creator1/3, Goto3/1  "FE_MOD_PWR"
  (0 device OFF / 1 ON)8/1(state) -> Bus Creator1/4, Goto6/1  "CHG_MOD_PWR"
  (0 device OFF / 1 ON)11/1(state) -> Bus Creator1/5, Goto11/1  "LD_MOD_PWR"
  Bus Selector2/2 -> (0 device OFF / 1 ON)12/2(DSBL)  "<MB_droop_DSBL>"
  Bus Selector2/1 -> (0 device OFF / 1 ON)12/1(EN)  "<MB_droop_EN>"
  Bus Selector2/4 -> (0 device OFF / 1 ON)13/2(DSBL)  "<SB_droop_DSBL>"
  Bus Selector2/3 -> (0 device OFF / 1 ON)13/1(EN)  "<SB_droop_EN>"
  Bus Selector2/6 -> (0 device OFF / 1 ON)14/2(DSBL)  "<FE_droop_DSBL>"
  Bus Selector2/5 -> (0 device OFF / 1 ON)14/1(EN)  "<FE_droop_EN>"
  Bus Selector2/8 -> (0 device OFF / 1 ON)15/2(DSBL)  "<CHG_droop_DSBL>"
  Bus Selector2/7 -> (0 device OFF / 1 ON)15/1(EN)  "<CHG_droop_EN>"
  Bus Selector2/10 -> (0 device OFF / 1 ON)16/2(DSBL)  "<LD_droop_DSBL>"
  Bus Selector2/9 -> (0 device OFF / 1 ON)16/1(EN)  "<LD_droop_EN>"
  (0 device OFF / 1 ON)14/1(state) -> Bus Creator/3  "FE_droop"
  (0 device OFF / 1 ON)15/1(state) -> Bus Creator/4  "CHG_droop"
  (0 device OFF / 1 ON)16/1(state) -> Bus Creator/5  "LD_droop"
  (0 device OFF / 1 ON)13/1(state) -> Bus Creator/2  "SB_droop"
  (0 device OFF / 1 ON)12/1(state) -> Bus Creator/1  "MB_droop"
  Bus Creator/1 -> [active_droop_bus]
  Bus Creator1/1 -> [device_power_on_bus]

== system BugE_v0_40_MAS_loads_reg/Master Controller/System Health ==
  Device-sent faults : Subsystem
  Internally detected faults : Subsystem
  Logical Operator : Logic  Operator=OR  AllPortsSameDT=off  OutDataTypeStr=boolean
  MB current limits : Subsystem
  SB current limits : Subsystem
  SM_FD_flag : Terminator
  e_stop_bus : Terminator
  internal_faults_bus : Terminator
  tag scope: MB_Imax=global, MB_Imin=global, SB_Imax=global, SB_Imin=global
  wires:
  Logical Operator/1 -> SM_FD_flag/1
  [devices_ON_bus] -> Device-sent faults/1(devices_ON), Internally detected faults/1(devices_ON)
  Device-sent faults/1(Bus (...)_e-stop) -> e_stop_bus/1
  Internally detected faults/2(Bus (...)_ms) -> internal_faults_bus/1
  MB current limits/1(I maximums) -> [MB_Imax]
  SB current limits/1(I maximums) -> [SB_Imax]
  SB current limits/2(I minimums) -> [SB_Imin]
  MB current limits/2(I minimums) -> [MB_Imin]
  Device-sent faults/2(FD) -> Logical Operator/1
  Internally detected faults/1(FD) -> Logical Operator/2
